simulink library "AccumulatorLIB"  (R2019a)
settings: Solver=VariableStepAuto  StartTime=0.0  StopTime=10.0  RelTol=1e-3
libraries: fl_lib x2, ee_lib x1, nesl_utility x1
settings Model: Creator=plewi  LastModifiedBy=plewi

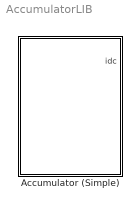
== system AccumulatorLIB ==
  Accumulator (Simple) : Subsystem  mask(Accumulator (Simple)){Vnom=450, R1=0.001, charge=7000}
      mask prompts: Vnom "Nominal voltage"; R1 "Internal resistance"; charge "Initial Charge"
      mask help: Simple battery model to represent the charge present in the accumulator.
      mask TypeOptions Vnom: Battery/Vnom
      mask TypeOptions R1: Battery/R1
      mask TypeOptions charge: Battery/charge

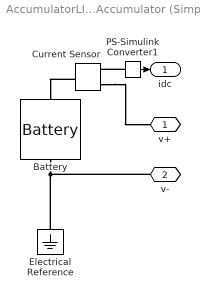
== system AccumulatorLIB/Accumulator (Simple) ==
  Battery : ee_lib/Sources/Battery  Vnom=Vnom V  R1=R1 Ohm  prm_AH=1  AH=14000 hr*A  V1=470 V  AH1=5000 hr*A  prm_R2=1  R2=inf Ohm  prm_dyn=1  Rp1=0.005 Ohm  tau1=30 s  Rp2=0.005 Ohm  tau2=30 s  Rp3=0.005 Ohm  tau3=30 s  Rp4=0.005 Ohm  tau4=30 s  Rp5=0.005 Ohm  tau5=30 s  prm_fade=1  N_fade=100  AH_fade=45 hr*A  R1_fade=2.02 Ohm  V1_fade=10.35 V  i_specify=on  i_priority=High  i=0 A  i_nominal_specify=off  i_nominal_unit=A  i_nominal_value=1  v_specify=off  v_priority=None  v=0 V  v_nominal_specify=off  v_nominal_unit=V  v_nominal_value=1  charge_specify=on  charge_priority=High  charge=charge hr*A  charge_nominal_specify=off  charge_nominal_unit=hr*A  charge_nominal_value=1  num_cycles_specify=off  num_cycles_priority=High  num_cycles=0  num_cycles_nominal_specify=off  num_cycles_nominal_unit=1  num_cycles_nominal_value=1  thermal_mass=30000 J/K  Tmeas=298.15 K  Vnom_T2=12 V  R1_T2=2.2 Ohm  V1_T2=11.4 V  R2_T2=2200 Ohm  Rp1_T2=0.005 Ohm  tau1_T2=30 s  Rp2_T2=0.005 Ohm  tau2_T2=30 s  Rp3_T2=0.005 Ohm  tau3_T2=30 s  Rp4_T2=0.005 Ohm  tau4_T2=30 s  Rp5_T2=0.005 Ohm  tau5_T2=30 s  Tmeas2=273.15 K  temperature_specify=off  temperature_priority=High  temperature=298.15 K  temperature_nominal_specify=off  temperature_nominal_unit=K  temperature_nominal_value=1
      settings: SourceProductName=Simscape Electrical
  Current Sensor : fl_lib/Electrical/Electrical Sensors/Current Sensor
  Electrical Reference : fl_lib/Electrical/Electrical Elements/Electrical Reference
      settings: SourceProductName=Foundation Library
  PS-Simulink Converter1 : nesl_utility/PS-Simulink Converter  PhysicalDomain=network_engine_domain  SubClassName=ps_output  LeftPortType=input  RightPortType=output  PseudoPeriodic=off  Frequencies=[]  Unit=1  AffineConversion=off
  v+ : PMIOPort  Side=Right
  v- : PMIOPort  Port=2  Side=Right
  idc : Outport
  wires:
  PS-Simulink Converter1/1 -> idc/1
  connections:
  Battery/RConn1 -- v-/RConn1 -- Electrical Reference/LConn1
  Current Sensor/LConn1 -- Battery/LConn1
  Current Sensor/RConn2 -- v+/RConn1
  PS-Simulink Converter1/LConn1 -- Current Sensor/RConn1
